simulink model "feedforward"  (R2023b)
settings: Solver=VariableStepAuto  StartTime=0.0  StopTime=10.0  RelTol=1e-3
settings Model: Creator=dzxion_microsoft  LastModifiedBy=dzxion_microsoft

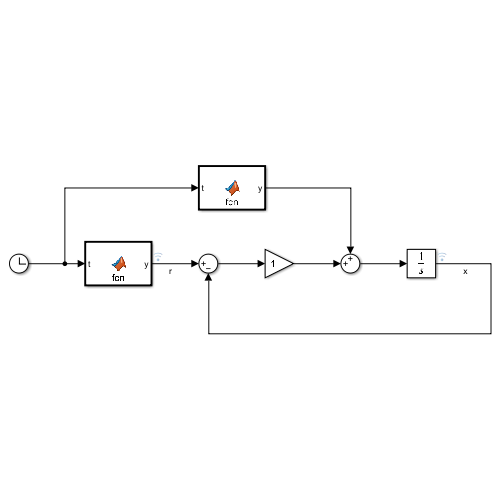
[thumbnail: Simulink's stored preview of the top-level diagram]
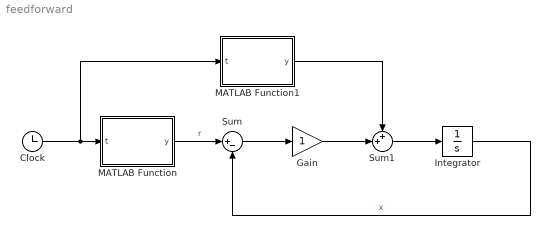
== system feedforward ==
  Clock : Clock
  Gain : Gain
  Integrator : Integrator
  MATLAB Function : MATLAB Function  TreatAsAtomicUnit=on
  MATLAB Function1 : MATLAB Function  TreatAsAtomicUnit=on
  Sum : Sum  Inputs=|+-
  Sum1 : Sum  Inputs=++|
  wires:
  Clock/1 -> MATLAB Function1/1(t), MATLAB Function/1(t)
  MATLAB Function/1(y) -> Sum/1  "r"
  Integrator/1 -> Sum/2  "x"
  Sum/1 -> Gain/1
  Gain/1 -> Sum1/2
  Sum1/1 -> Integrator/1
  MATLAB Function1/1(y) -> Sum1/1

== matlab function feedforward/MATLAB Function ==
  data: t input; y output
function y = fcn(t)

w = 1;
y = sin(w*t);

== matlab function feedforward/MATLAB Function1 ==
  data: t input; y output
function y = fcn(t)

w = 1;
y = cos(w*t);
